simulink model "single_pendulum"  (R2022a)
settings: Solver=VariableStepAuto  StartTime=0.0  StopTime=10  RelTol=1e-8
values from neighbouring files (symbols this model uses):
  k = [-9.21108429178e-06 -0.000351785194902 -1384.51415715 -3.88080147723]    [kval.mat]
settings Model: Creator=natha  LastModifiedBy=natha
settings DebuggingCC: UnconnectedInputMsg=warning  UnconnectedOutputMsg=warning  UnconnectedLineMsg=warning
settings RTWCC: DLArmComputeVersion=19.05

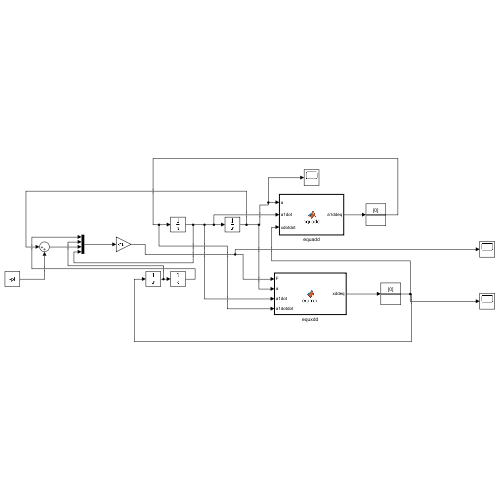
[thumbnail: Simulink's stored preview of the top-level diagram]
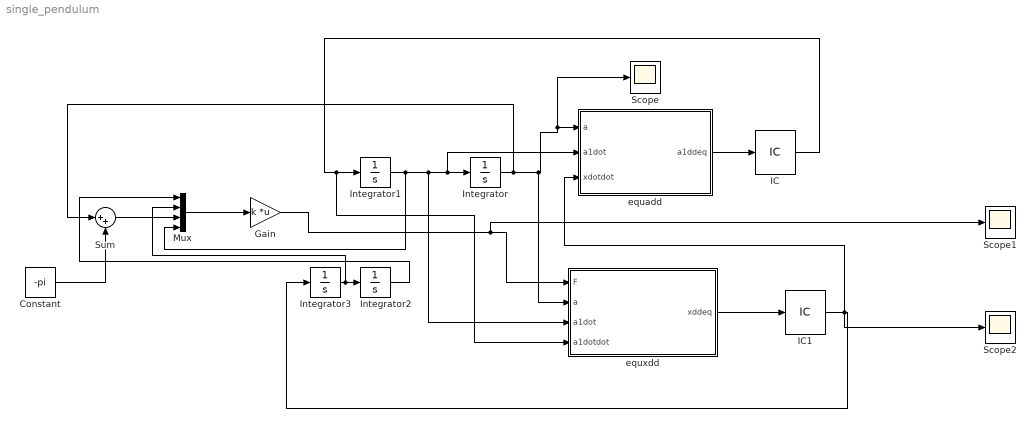
== system single_pendulum ==
  Constant : Constant  Value=-pi
  Gain : Gain  Gain=k  Multiplication=Matrix(K*u)
  IC : InitialCondition  Value=0
  IC1 : InitialCondition  Value=0
  Integrator : Integrator  InitialCondition=pi+0.05
  Integrator1 : Integrator
  Integrator2 : Integrator
  Integrator3 : Integrator
  Mux : Mux
  Scope : Scope
  Scope1 : Scope
  Scope2 : Scope
  Sum : Sum  Inputs=|++
  equadd : MATLAB Function  TreatAsAtomicUnit=on
  equxdd : MATLAB Function  TreatAsAtomicUnit=on
  wires:
  Integrator1/1 -> Mux/4, equxdd/3(a1dot), equadd/2(a1dot), Integrator/1
  Integrator3/1 -> Mux/2, Integrator2/1
  equxdd/1(xddeq) -> IC1/1
  equadd/1(a1ddeq) -> IC/1
  IC/1 -> equxdd/4(a1dotdot), Integrator1/1
  Integrator/1 -> Sum/1, equxdd/2(a), Scope/1, equadd/1(a)
  IC1/1 -> equadd/3(xdotdot), Scope2/1, Integrator3/1
  Integrator2/1 -> Mux/1
  Mux/1 -> Gain/1
  Constant/1 -> Sum/2
  Sum/1 -> Mux/3
  Gain/1 -> Scope1/1, equxdd/1(F)

== matlab function single_pendulum/equxdd ==
  data: F input; xddeq output; a input; a1dot input; a1dotdot input
function xddeq = equxdd(F,a,a1dot,a1dotdot)
%#codegen

%    This function was generated by the Symbolic Math Toolbox version 9.1.
%    11-Apr-2022 11:59:45

xddeq = F.*(2.0e+2./7.1e+1)-a1dotdot.*cos(a).*4.091549295774648e-2+a1dot.^2.*sin(a).*4.091549295774648e-2;

== matlab function single_pendulum/equadd ==
  data: a input; a1dot input; a1ddeq output; xdotdot input
function a1ddeq = equadd(a,a1dot,xdotdot)
%#codegen

%    This function was generated by the Symbolic Math Toolbox version 9.1.
%    11-Apr-2022 11:59:44

t2 = cos(a);
t3 = sin(a);
t4 = a1dot.^2;
a1ddeq = -(a1dot.*1.54e-3+t3.*1.42345e-1+t2.*(xdotdot-t3.*t4.*(7.0./4.0e+1)).*1.4525e-2+t2.*t3.*t4.*2.541875e-3)./(t2.^2.*2.541875e-3+t3.^2.*2.541875e-3+8.517540233333332e-4);
